simulink model "E01"  (R2014a)
settings: Solver=ode45  StartTime=0.0  StopTime=200  RelTol=1e-3
values from neighbouring files (symbols this model uses):
  Kr = 1    [E01.m]
libraries: cstblocks x2
settings Model: Creator=Davide  LastModifiedBy=Davide

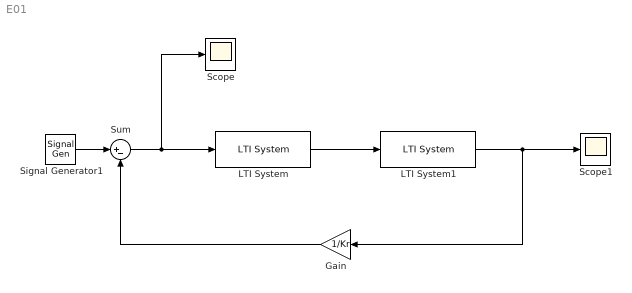
== system E01 ==
  Gain : Gain  Gain=1/Kr
  LTI System : cstblocks/LTI System  sys=C  IC=[]
  LTI System1 : cstblocks/LTI System  sys=F  IC=[]
  Scope : Scope
  Scope1 : Scope
  Signal Generator1 : SignalGenerator  Frequency=0.1  Units=rad/sec
  Sum : Sum  Inputs=|+-
  wires:
  LTI System/1 -> LTI System1/1
  Signal Generator1/1 -> Sum/1
  Gain/1 -> Sum/2
  LTI System1/1 -> Gain/1, Scope1/1
  Sum/1 -> Scope/1, LTI System/1
